simulink model "IKTrajectoryControlExamplechangepoints_MechanicalArm"  (R2019b)
settings: Solver=ode3  StartTime=0.0  StopTime=10  FixedStep=Ts  RelTol=1e-3
PostLoadFcn:
  | robot=importrobot('demo.urdf');
  | robot.DataFormat = 'column';
  | 
  | I = imread('coins.png');
  | imageOrigin = [40,20,0.08];
  | scale = .15;
model workspace (MAT data in the model file):
  I = [49 47 48 48 48 48 48 51 50 51 50 47 ... (73800 elements, 246x300)]
  Ts = 0.01
  filterConst = 0.08
  force_range = [0.8 0.9]
  imageOrigin = [0.4 0.2 0.08]
  initTargetPose = [-1 0 -1.22464679915e-16 0 0 1 0 0 1.22464679915e-16 0 -1 0 ... (16 elements, 4x4)]
  q0 = [0.422405030154; 0; -1.22880122285; 0]
  robot : robotics.RigidBodyTree (value not decoded)
  scale = 0.0015
  wayPoints = [0 0 0 0 0 0 0 0 0 0 0 0 ... (1212 elements, 202x6)]
  weights = [1 1 1 1]
  weights1 = [1 1 1 1 1 1]
undefined symbols (not defined in the file or in its folder): Levenberg, Marquardt
libraries: robotmaniplib x6, simulink x2
(part 2 of 2)

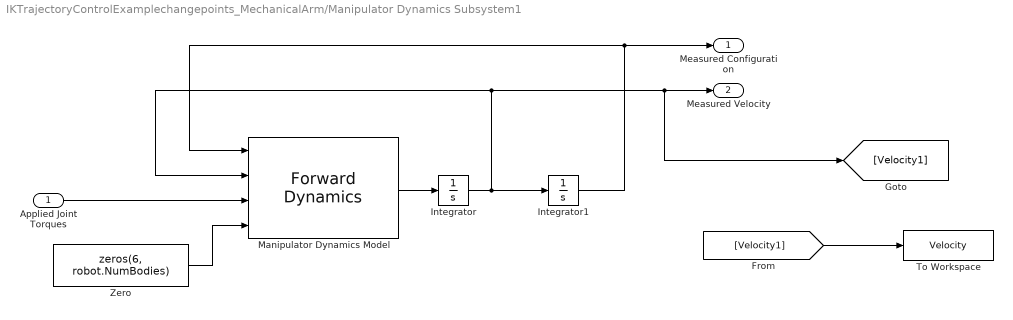
== system IKTrajectoryControlExamplechangepoints_MechanicalArm/Manipulator Dynamics Subsystem1 ==
  Applied Joint Torques : Inport
  Integrator : Integrator
  Integrator1 : Integrator  InitialCondition=q0
  Manipulator Dynamics Model : robotmaniplib/Forward Dynamics  RigidBodyTree=robot  SimulateUsing=Interpreted execution
      settings: SourceProductName=Robotics System Toolbox
  To Workspace : ToWorkspace  VariableName=Velocity  SaveFormat=Timeseries  SampleTime=-1
  Zero : Constant  Value=zeros(6, robot.NumBodies)  OutDataTypeStr=Inherit: Inherit via back propagation
  Measured Configuration : Outport  VectorParamsAs1DForOutWhenUnconnected=off
  Measured Velocity : Outport  Port=2  VectorParamsAs1DForOutWhenUnconnected=off
  wires:
  Integrator1/1 -> Manipulator Dynamics Model/1, Measured Configuration/1
  Manipulator Dynamics Model/1 -> Integrator/1
  Integrator/1 -> Integrator1/1, Manipulator Dynamics Model/2, [Velocity1], Measured Velocity/1
  Applied Joint Torques/1 -> Manipulator Dynamics Model/3
  Zero/1 -> Manipulator Dynamics Model/4
  [Velocity1] -> To Workspace/1

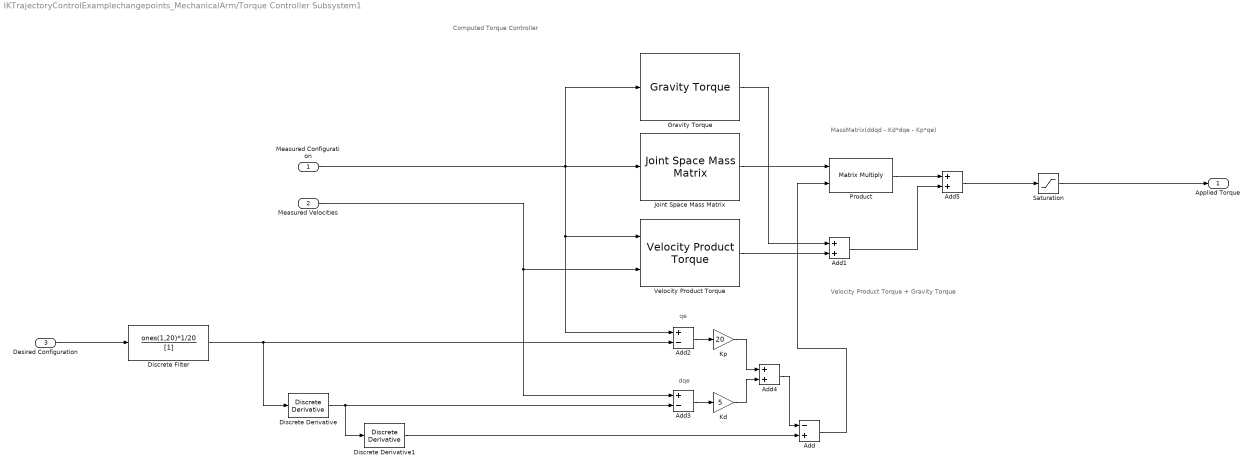
== system IKTrajectoryControlExamplechangepoints_MechanicalArm/Torque Controller Subsystem1 ==
  note: Computed Torque Controller
  note: MassMatrix(ddqd - Kd*dqe - Kp*qe)
  note: Velocity Product Torque + Gravity Torque
  note: dqe
  note: qe
  Measured Configuration : Inport
  Measured Velocities : Inport  Port=2
  Desired Configuration : Inport  Port=3
  Add : Sum  Inputs=-+
  Add1 : Sum
  Add2 : Sum  Inputs=+-
  Add3 : Sum  Inputs=+-
  Add4 : Sum
  Add5 : Sum
  Discrete Derivative : simulink/Discrete/Discrete Derivative  gainval=1.0  ICPrevScaledInput=0.0  OutMin=[]  OutMax=[]  OutDataType=fixdt(1, 16)  OutScaling=2^-10  DoSatur=off
  Discrete Derivative1 : simulink/Discrete/Discrete Derivative  gainval=1.0  ICPrevScaledInput=0.0  OutMin=[]  OutMax=[]  OutDataType=fixdt(1, 16)  OutScaling=2^-10  DoSatur=off
  Discrete Filter : DiscreteFilter  Numerator=ones(1,20)*1/20  Denominator=[1]  InitialStates=repmat(q0',19,1)
  Gravity Torque : robotmaniplib/Gravity Torque  RigidBodyTree=robot  SimulateUsing=Interpreted execution
      settings: SourceProductName=Robotics System Toolbox
  Joint Space Mass Matrix : robotmaniplib/Joint Space Mass Matrix  RigidBodyTree=robot  SimulateUsing=Interpreted execution
      settings: SourceProductName=Robotics System Toolbox
  Kd : Gain  Gain=5
  Kp : Gain  Gain=20
  Product : Product  Multiplication=Matrix(*)
  Saturation : Saturate  UpperLimit=100  LowerLimit=-100
  Velocity Product Torque : robotmaniplib/Velocity Product Torque  RigidBodyTree=robot  SimulateUsing=Interpreted execution
      settings: SourceProductName=Robotics System Toolbox  SourceProductBaseCode=RO
  Applied Torque : Outport  VectorParamsAs1DForOutWhenUnconnected=off
  wires:
  Saturation/1 -> Applied Torque/1
  Velocity Product Torque/1 -> Add1/2
  Gravity Torque/1 -> Add1/1
  Add1/1 -> Add5/2
  Product/1 -> Add5/1
  Add5/1 -> Saturation/1
  Kd/1 -> Add4/2
  Kp/1 -> Add4/1
  Add3/1 -> Kd/1
  Add2/1 -> Kp/1
  Discrete Derivative/1 -> Add3/2, Discrete Derivative1/1
  Desired Configuration/1 -> Discrete Filter/1
  Add/1 -> Product/2
  Discrete Derivative1/1 -> Add/2
  Add4/1 -> Add/1
  Measured Velocities/1 -> Velocity Product Torque/2, Add3/1
  Measured Configuration/1 -> Add2/1, Velocity Product Torque/1, Gravity Torque/1, Joint Space Mass Matrix/1
  Joint Space Mass Matrix/1 -> Product/1
  Discrete Filter/1 -> Discrete Derivative/1, Add2/2

== matlab function IKTrajectoryControlExamplechangepoints_MechanicalArm/MATLAB Function2 ==
  data: u input; fn output; ft output
function [fn,ft] = fcn(u)
%#codegen
point = zeros(100,3);
fn = zeros(100,3);
ft = zeros(100,3);

for i = 1 : 100
    point(i,1) = 0;
    point(i,2) = -1+0.02*i;
    point(i,3) = sqrt(1-point(i,2)*point(i,2));
    
    fn(i,1) = 0;
    fn(i,2) = 0-point(i,2);
    fn(i,3) = 0-point(i,3);
    ft(i,2:3) = fn(i,2:3)*[0  1
                          -1 0];

end

% for i = 1 : 100
%     point(i,1) = 0;
%     point(i,2) = -1.57+0.0314*i;
%     point(i,3) = -cos(point(i,2));
%     fn(i,1) = 0;
%     fn(i,2) = 0-point(i,2);
%     fn(i,3) = 0-point(i,3);
%     ft(i,2:3) = fn(i,2:3)*[0  -1
%                            1  0];
% 
% end

== matlab function IKTrajectoryControlExamplechangepoints_MechanicalArm/MATLAB Function ==
  data: fn input; ft input; targetPose output; currentPose input
function targetPose  = fcn(fn, ft, currentPose)  
   
   k = 0.01;
%    targetPose = zeros(3,1);
%    currentPose = zeros(3,1);
   u = zeros(3,1);
   q = zeros(3,1);
   q = currentPose;
   persistent i;
   if isempty(i)
      i = 1;
   end

%    if i == 1
%        q = [0;-1;0];
%    end
   
   f1 = normest(fn(i,:));
   f2 = normest(ft(i,:));
   if f1 < 0
     u(1,1) = q(1,end)+k*fn(i,1)/f1;
     u(2,1) = q(2,end)+k*fn(i,2)/f1;
     u(3,1) = q(3,end)+k*fn(i,3)/f1;
   elseif f1 >= 0 && f1 < 10 
     u(1,1) = q(1,end)+k*ft(i,1)/f2;
     u(2,1) = q(2,end)+k*ft(i,2)/f2;
     u(3,1) = q(3,end)+k*ft(i,3)/f2;
   elseif f1 >= 10
     u(1,1) = q(1,end)-k*fn(i,1)/f1;
     u(2,1) = q(2,end)-k*fn(i,2)/f1;
     u(3,1) = q(3,end)-k*fn(i,3)/f1;
   end
   
   TP = eul2tform([0,0,0]);   %欧拉角转旋转矩阵
   TP(1:3,end) = u(1:3,1); 
   
   i = i+1;
 
   targetPose = TP;

== matlab function IKTrajectoryControlExamplechangepoints_MechanicalArm/MATLAB Function1 ==
  data: currentPose input; targetPose input
function waypointTracking(currentPose, targetPose)
%#codegen

% persistent f1 a1
% 
% if isempty(f1)
%     f1 = figure;
%     title('Waypoint Tracking-force');
%     a1 = axes;
%     axis(a1, [-2,2, -2,2, -2,2]);
%     set(f1, 'Visible', 'on');
% end

targetPoint = targetPose(1:3,end);
currentPoint = currentPose(1:3,end);


plot3(targetPoint(1), targetPoint(2), targetPoint(3), 'go', 'MarkerSize', 5);
hold on;
plot3(currentPoint(1), currentPoint(2), currentPoint(3), 'ro', 'MarkerSize', 5);
